simulink model "liftsubsystem"  (R2025b)
settings: Solver=VariableStepAuto  StartTime=0.0  StopTime=10  RelTol=1e-3
values from neighbouring files (symbols this model uses):
  N = 20    [ocp_arm.m]
undefined symbols (not defined in the file or in its folder): lx, ly, lz, M, m_w, X, Y, Z
libraries: sm_lib x138, nesl_utility x30, sharedTrackingLibrary x6, slpidlib x3, simulink x3, eeSlidingModeController x1, robotcorelib x1
(part 1 of 4)
settings Model: Creator=itsan  LastModifiedBy=itsan

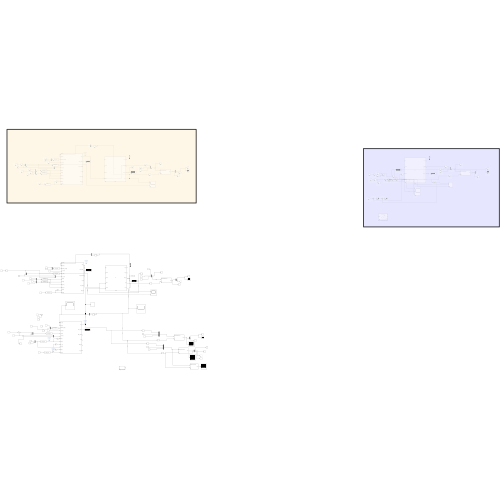
[thumbnail: Simulink's stored preview of the top-level diagram]
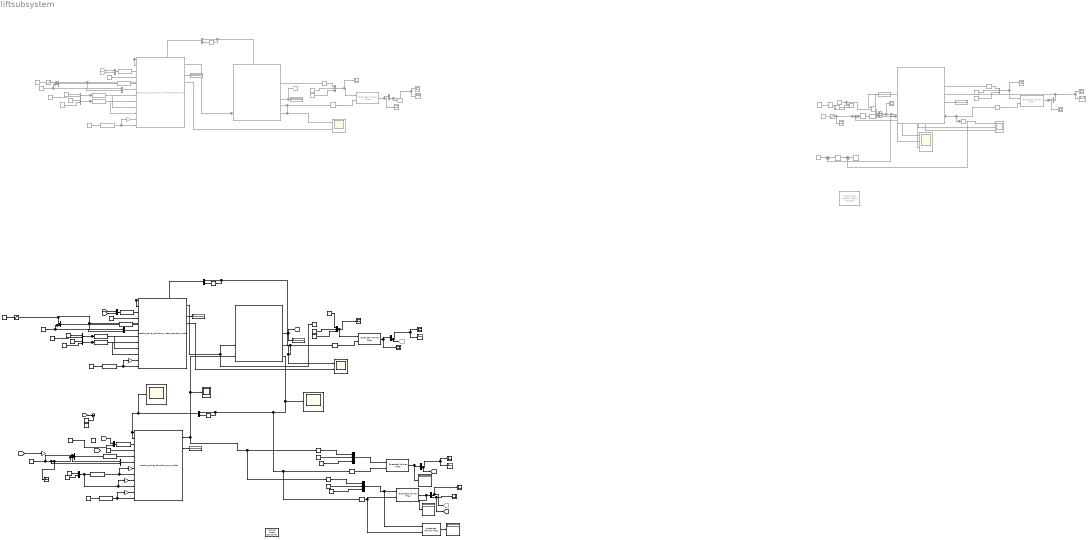
== system liftsubsystem ==
  note: Lift
  Constant : Constant  Commented=on  Value=0.5
  Constant1 : Constant  Commented=on  Value=9.81
  Constant10 : Constant  Commented=on  Value=0.01
  Constant11 : Constant  Commented=on  Value=0.5
  Constant12 : Constant  Commented=on  Value=0.8
  Constant13 : Constant  Commented=on  Value=0
  Constant14 : Constant  Commented=on  Value=150
  Constant{15,26,34..35} (4 alike) : Constant  Value=0.01
  Constant16 : Constant  Value=0.5
  Constant17 : Constant  Value=0.8
  Constant18 : Constant  Value=0
  Constant19 : Constant  Value=150
  Constant2 : Constant  Commented=on  Value=12
  Constant20 : Constant  Value=[0 0 0]
  Constant21 : Constant  Value=-0.5
  Constant22 : Constant  Value=0
  Constant23 : Constant  Value=0.43
  Constant24 : Constant  Value=0.5
  Constant25 : Constant  Value=0.5
  Constant27 : Constant  Value=100
  Constant28 : Constant  Value=[0 0 0]
  Constant29 : Constant  Value=7
  Constant3 : Constant  Commented=on  Value=0.43
  Constant30 : Constant  Value=0
  Constant31 : Constant  Value=0.4
  Constant{32..33,36..37} (4 alike) : Constant  Value=5
  Constant4 : Constant  Commented=on  Value=0.01
  Constant5 : Constant  Commented=on  Value=0.43
  Constant6 : Constant  Commented=on  Value=[0 0 0]
  Constant7 : Constant  Commented=on  Value=-0.5
  Constant8 : Constant  Commented=on  Value=0
  Constant9 : Constant  Commented=on  Value=0.43
  Cos : Trigonometry  Commented=on  Operator=cos
  Demux : Demux  Commented=on  Outputs=3
  Demux1 : Demux  Commented=on  Outputs=3
  Demux2 : Demux  Outputs=3
  Demux3 : Demux  Outputs=3
  Demux4 : Demux
  Derivative : Derivative  Commented=on
  Derivative1 : Derivative  Commented=on
  Derivative2 : Derivative
  Derivative3 : Derivative
  Display{,1..5} (6 alike) : Display  Commented=on
  Display{6..13} (8 alike) : Display
  Divide : Product  Commented=on  Inputs=***
  Divide1 : Product  Commented=on  Inputs=**
  Extended Kalman Filter : sharedTrackingLibrary/Extended Kalman Filter  Commented=on  StateTransitionFcn=myStateTransitionFcn  HasStateTransitionJacobianFcn=off  HasAdditiveProcessNoise=Additive  ProcessNoise=diag([1e-6, 1e-4, 1e-8])  HasTimeVaryingProcessNoise=off  HasStateTransitionFcnExtraArgument=1  InitialState=[0; 0; 10]  InitialStateCovariance=diag([1e-2, 1e-2, 100])  MeasurementFcn1=myMeasurementFcn  HasMeasurementJacobianFcn1=off  HasMeasurementEnablePort1=off  HasAdditiveMeasurementNoise1=Additive  MeasurementNoise1=diag([1e-2])  HasTimeVaryingMeasurementNoise1=off  HasMeasurementFcnExtraArgument1=0  HasMeasurementWrapping1=off  MeasurementFcn2=myMeasurementFcn  HasMeasurementJacobianFcn2=off  HasMeasurementEnablePort2=off  HasAdditiveMeasurementNoise2=Additive  MeasurementNoise2=1  HasTimeVaryingMeasurementNoise2=off  HasMeasurementFcnExtraArgument2=0  HasMeasurementWrapping2=off  MeasurementFcn3=myMeasurementFcn  HasMeasurementJacobianFcn3=off  HasMeasurementEnablePort3=off  HasAdditiveMeasurementNoise3=Additive  MeasurementNoise3=1  HasTimeVaryingMeasurementNoise3=off  HasMeasurementFcnExtraArgument3=0  HasMeasurementWrapping3=off  MeasurementFcn4=myMeasurementFcn  HasMeasurementJacobianFcn4=off  HasMeasurementEnablePort4=off  HasAdditiveMeasurementNoise4=Additive  MeasurementNoise4=1  HasTimeVaryingMeasurementNoise4=off  HasMeasurementFcnExtraArgument4=0  HasMeasurementWrapping4=off  MeasurementFcn5=myMeasurementFcn  HasMeasurementJacobianFcn5=off  HasMeasurementEnablePort5=off  HasAdditiveMeasurementNoise5=Additive  MeasurementNoise5=1  HasTimeVaryingMeasurementNoise5=off  HasMeasurementFcnExtraArgument5=0  HasMeasurementWrapping5=off  EnableMultirate=off  StateTransitionFcnSampleTime=1  MeasurementFcn1SampleTime=1  MeasurementFcn2SampleTime=1  MeasurementFcn3SampleTime=1  MeasurementFcn4SampleTime=1  MeasurementFcn5SampleTime=1  UseCurrentEstimator=on  OutputStateCovariance=off  DataType=double  SampleTime=0.01  NumberOfMeasurements=1
  Extended Kalman Filter1 : sharedTrackingLibrary/Extended Kalman Filter  Commented=on  StateTransitionFcn=myStateTransitionFcn  HasStateTransitionJacobianFcn=off  HasAdditiveProcessNoise=Additive  ProcessNoise=diag([1e-6, 1e-4, 1e-8])  HasTimeVaryingProcessNoise=off  HasStateTransitionFcnExtraArgument=1  InitialState=[0; 0; 10]  InitialStateCovariance=diag([1e-2, 1e-2, 100])  MeasurementFcn1=myMeasurementFcn  HasMeasurementJacobianFcn1=off  HasMeasurementEnablePort1=off  HasAdditiveMeasurementNoise1=Additive  MeasurementNoise1=diag([1e-2])  HasTimeVaryingMeasurementNoise1=off  HasMeasurementFcnExtraArgument1=0  HasMeasurementWrapping1=off  MeasurementFcn2=myMeasurementFcn  HasMeasurementJacobianFcn2=off  HasMeasurementEnablePort2=off  HasAdditiveMeasurementNoise2=Additive  MeasurementNoise2=1  HasTimeVaryingMeasurementNoise2=off  HasMeasurementFcnExtraArgument2=0  HasMeasurementWrapping2=off  MeasurementFcn3=myMeasurementFcn  HasMeasurementJacobianFcn3=off  HasMeasurementEnablePort3=off  HasAdditiveMeasurementNoise3=Additive  MeasurementNoise3=1  HasTimeVaryingMeasurementNoise3=off  HasMeasurementFcnExtraArgument3=0  HasMeasurementWrapping3=off  MeasurementFcn4=myMeasurementFcn  HasMeasurementJacobianFcn4=off  HasMeasurementEnablePort4=off  HasAdditiveMeasurementNoise4=Additive  MeasurementNoise4=1  HasTimeVaryingMeasurementNoise4=off  HasMeasurementFcnExtraArgument4=0  HasMeasurementWrapping4=off  MeasurementFcn5=myMeasurementFcn  HasMeasurementJacobianFcn5=off  HasMeasurementEnablePort5=off  HasAdditiveMeasurementNoise5=Additive  MeasurementNoise5=1  HasTimeVaryingMeasurementNoise5=off  HasMeasurementFcnExtraArgument5=0  HasMeasurementWrapping5=off  EnableMultirate=off  StateTransitionFcnSampleTime=1  MeasurementFcn1SampleTime=1  MeasurementFcn2SampleTime=1  MeasurementFcn3SampleTime=1  MeasurementFcn4SampleTime=1  MeasurementFcn5SampleTime=1  UseCurrentEstimator=on  OutputStateCovariance=off  DataType=double  SampleTime=0.01  NumberOfMeasurements=1
  Extended Kalman Filter2 : sharedTrackingLibrary/Extended Kalman Filter  StateTransitionFcn=liftStateTransitionFcn  HasStateTransitionJacobianFcn=off  HasAdditiveProcessNoise=Additive  ProcessNoise=diag([1e-6, 1e-4, 1e-8])  HasTimeVaryingProcessNoise=off  HasStateTransitionFcnExtraArgument=1  InitialState=[0; 0; 10]  InitialStateCovariance=diag([1e-2, 1e-2, 100])  MeasurementFcn1=liftMeasurementFcn  HasMeasurementJacobianFcn1=off  HasMeasurementEnablePort1=off  HasAdditiveMeasurementNoise1=Additive  MeasurementNoise1=diag([1e-2])  HasTimeVaryingMeasurementNoise1=off  HasMeasurementFcnExtraArgument1=0  HasMeasurementWrapping1=off  MeasurementFcn2=myMeasurementFcn  HasMeasurementJacobianFcn2=off  HasMeasurementEnablePort2=off  HasAdditiveMeasurementNoise2=Additive  MeasurementNoise2=1  HasTimeVaryingMeasurementNoise2=off  HasMeasurementFcnExtraArgument2=0  HasMeasurementWrapping2=off  MeasurementFcn3=myMeasurementFcn  HasMeasurementJacobianFcn3=off  HasMeasurementEnablePort3=off  HasAdditiveMeasurementNoise3=Additive  MeasurementNoise3=1  HasTimeVaryingMeasurementNoise3=off  HasMeasurementFcnExtraArgument3=0  HasMeasurementWrapping3=off  MeasurementFcn4=myMeasurementFcn  HasMeasurementJacobianFcn4=off  HasMeasurementEnablePort4=off  HasAdditiveMeasurementNoise4=Additive  MeasurementNoise4=1  HasTimeVaryingMeasurementNoise4=off  HasMeasurementFcnExtraArgument4=0  HasMeasurementWrapping4=off  MeasurementFcn5=myMeasurementFcn  HasMeasurementJacobianFcn5=off  HasMeasurementEnablePort5=off  HasAdditiveMeasurementNoise5=Additive  MeasurementNoise5=1  HasTimeVaryingMeasurementNoise5=off  HasMeasurementFcnExtraArgument5=0  HasMeasurementWrapping5=off  EnableMultirate=off  StateTransitionFcnSampleTime=1  MeasurementFcn1SampleTime=1  MeasurementFcn2SampleTime=1  MeasurementFcn3SampleTime=1  MeasurementFcn4SampleTime=1  MeasurementFcn5SampleTime=1  UseCurrentEstimator=on  OutputStateCovariance=off  DataType=double  SampleTime=0.01  NumberOfMeasurements=1
  Extended Kalman Filter3 : sharedTrackingLibrary/Extended Kalman Filter  StateTransitionFcn=armStateTransitionFcn  HasStateTransitionJacobianFcn=off  HasAdditiveProcessNoise=Additive  ProcessNoise=diag([1e-8, 1e-6,1e-10])  HasTimeVaryingProcessNoise=off  HasStateTransitionFcnExtraArgument=1  InitialState=[0;0;0.3]  InitialStateCovariance=diag([1e-4, 1e-4,100])  MeasurementFcn1=armMeasurementFcn  HasMeasurementJacobianFcn1=off  HasMeasurementEnablePort1=off  HasAdditiveMeasurementNoise1=Additive  MeasurementNoise1=1e-4  HasTimeVaryingMeasurementNoise1=off  HasMeasurementFcnExtraArgument1=0  HasMeasurementWrapping1=off  MeasurementFcn2=myMeasurementFcn  HasMeasurementJacobianFcn2=off  HasMeasurementEnablePort2=off  HasAdditiveMeasurementNoise2=Additive  MeasurementNoise2=1  HasTimeVaryingMeasurementNoise2=off  HasMeasurementFcnExtraArgument2=0  HasMeasurementWrapping2=off  MeasurementFcn3=myMeasurementFcn  HasMeasurementJacobianFcn3=off  HasMeasurementEnablePort3=off  HasAdditiveMeasurementNoise3=Additive  MeasurementNoise3=1  HasTimeVaryingMeasurementNoise3=off  HasMeasurementFcnExtraArgument3=0  HasMeasurementWrapping3=off  MeasurementFcn4=myMeasurementFcn  HasMeasurementJacobianFcn4=off  HasMeasurementEnablePort4=off  HasAdditiveMeasurementNoise4=Additive  MeasurementNoise4=1  HasTimeVaryingMeasurementNoise4=off  HasMeasurementFcnExtraArgument4=0  HasMeasurementWrapping4=off  MeasurementFcn5=myMeasurementFcn  HasMeasurementJacobianFcn5=off  HasMeasurementEnablePort5=off  HasAdditiveMeasurementNoise5=Additive  MeasurementNoise5=1  HasTimeVaryingMeasurementNoise5=off  HasMeasurementFcnExtraArgument5=0  HasMeasurementWrapping5=off  EnableMultirate=off  StateTransitionFcnSampleTime=1  MeasurementFcn1SampleTime=1  MeasurementFcn2SampleTime=1  MeasurementFcn3SampleTime=1  MeasurementFcn4SampleTime=1  MeasurementFcn5SampleTime=1  UseCurrentEstimator=on  OutputStateCovariance=off  DataType=double  SampleTime=0.01  NumberOfMeasurements=1
  Extended Kalman Filter5 : sharedTrackingLibrary/Extended Kalman Filter  StateTransitionFcn=armMassStateTransitionFcn  HasStateTransitionJacobianFcn=off  HasAdditiveProcessNoise=Additive  ProcessNoise=diag([1e-8, 1e-6,1e-10,1e-10])  HasTimeVaryingProcessNoise=off  HasStateTransitionFcnExtraArgument=1  InitialState=[0;0;0.3;5]  InitialStateCovariance=diag([1e-4, 1e-4,100,100])  MeasurementFcn1=armMeasurementFcn  HasMeasurementJacobianFcn1=off  HasMeasurementEnablePort1=off  HasAdditiveMeasurementNoise1=Additive  MeasurementNoise1=1e-4  HasTimeVaryingMeasurementNoise1=off  HasMeasurementFcnExtraArgument1=0  HasMeasurementWrapping1=off  MeasurementFcn2=myMeasurementFcn  HasMeasurementJacobianFcn2=off  HasMeasurementEnablePort2=off  HasAdditiveMeasurementNoise2=Additive  MeasurementNoise2=1  HasTimeVaryingMeasurementNoise2=off  HasMeasurementFcnExtraArgument2=0  HasMeasurementWrapping2=off  MeasurementFcn3=myMeasurementFcn  HasMeasurementJacobianFcn3=off  HasMeasurementEnablePort3=off  HasAdditiveMeasurementNoise3=Additive  MeasurementNoise3=1  HasTimeVaryingMeasurementNoise3=off  HasMeasurementFcnExtraArgument3=0  HasMeasurementWrapping3=off  MeasurementFcn4=myMeasurementFcn  HasMeasurementJacobianFcn4=off  HasMeasurementEnablePort4=off  HasAdditiveMeasurementNoise4=Additive  MeasurementNoise4=1  HasTimeVaryingMeasurementNoise4=off  HasMeasurementFcnExtraArgument4=0  HasMeasurementWrapping4=off  MeasurementFcn5=myMeasurementFcn  HasMeasurementJacobianFcn5=off  HasMeasurementEnablePort5=off  HasAdditiveMeasurementNoise5=Additive  MeasurementNoise5=1  HasTimeVaryingMeasurementNoise5=off  HasMeasurementFcnExtraArgument5=0  HasMeasurementWrapping5=off  EnableMultirate=off  StateTransitionFcnSampleTime=1  MeasurementFcn1SampleTime=1  MeasurementFcn2SampleTime=1  MeasurementFcn3SampleTime=1  MeasurementFcn4SampleTime=1  MeasurementFcn5SampleTime=1  UseCurrentEstimator=on  OutputStateCovariance=off  DataType=double  SampleTime=0.01  NumberOfMeasurements=1
  From : From  Commented=on  GotoTag=Mass
  From1 : From  Commented=on  GotoTag=Pitch
  Gain : Gain  Commented=on  Gain=-1
  Gain{1..5} (5 alike) : Gain  Gain=-1
  Goto : Goto  Commented=on  GotoTag=Mass
  Goto1 : Goto  Commented=on  GotoTag=Pitch
  Goto2 : Goto  Commented=on  GotoTag=Mass
  Goto5 : Goto  Commented=on  GotoTag=rx
  Mux{,2,5..7} (5 alike) : Mux  Commented=on  Inputs=2
  Mux1 : Mux  Commented=on  Inputs=3
  Mux{8,10,12..15,18..20} (9 alike) : Mux  Inputs=2
  Mux{9,11,16..17,21} (5 alike) : Mux  Inputs=3
  Mux3 : Mux  Commented=on  Inputs=3
  Mux4 : Mux  Commented=on  Inputs=3
  PD : slpidlib/PID Controller  Commented=on  Controller=PID  Form=Parallel  TimeDomain=Continuous-time  UseExternalTs=off  SampleTime=-1  IntegratorMethod=Forward Euler  FilterMethod=Forward Euler  ControllerParametersSource=internal  P=1  I=0.001  UseKiTs=off  D=22  UseExternalDerivativeSource=off  N=15  UseFilter=on  TunerSelectOption=Transfer Function Based (PID Tuner App)  InitialConditionSource=internal  InitialConditionForIntegrator=0  InitialConditionForFilter=0  DifferentiatorICPrevScaledInput=0  ExternalReset=none  TrackingMode=off  Kt=1  LimitOutput=on  SatLimitsSource=internal  UpperSaturationLimit=100  LowerSaturationLimit=-100  LinearizeAsGain=on  AntiWindupMode=back-calculation  Kb=3  LimitIntegrator=off  UpperIntegratorSaturationLimit=inf  LowerIntegratorSaturationLimit=-inf  POutMin=[]  POutMax=[]  IOutMin=[]  IOutMax=[]  DOutMin=[]  DOutMax=[]  NOutMin=[]  NOutMax=[]  SumOutMin=[]  SumOutMax=[]  SaturationOutMin=[]  SaturationOutMax=[]  PParamMin=[]  PParamMax=[]  IParamMin=[]  IParamMax=[]  DParamMin=[]  DParamMax=[]  NParamMin=[]  NParamMax=[]  KbParamMin=[]  KbParamMax=[]  KtParamMin=[]  KtParamMax=[]  KbOutMin=[]  KbOutMax=[]  KtOutMin=[]  KtOutMax=[]  IntegratorOutMin=[]  IntegratorOutMax=[]  FilterOutMin=[]  FilterOutMax=[]  SumI1OutMin=[]  SumI1OutMax=[]  SumI2OutMin=[]  SumI2OutMax=[]  SumI3OutMin=[]  SumI3OutMax=[]  SumI4OutMin=[]  SumI4OutMax=[]  SumDOutMin=[]  SumDOutMax=[]  DifferentiatorOutMin=[]  DifferentiatorOutMax=[]  FilterDiffOutCoefMin=[]  FilterDiffOutCoefMax=[]  ReciprocalOutMin=[]  ReciprocalOutMax=[]  SumDenOutMin=[]  SumDenOutMax=[]  SumNumOutMin=[]  SumNumOutMax=[]  DivideOutMin=[]  DivideOutMax=[]  UdiffTsProdOutMin=[]  UdiffTsProdOutMax=[]  NTsProdOutMin=[]  NTsProdOutMax=[]  UintegralTsProdOutMin=[]  UintegralTsProdOutMax=[]  UngainTsProdOutMin=[]  UngainTsProdOutMax=[]  ClampingZeroOutDataTypeStr=Inherit: Inherit via back propagation  ClampingZeroOutMin=[]  ClampingZeroOutMax=[]  FilterDenConstantOutDataTypeStr=Inherit: Inherit via back propagation  FilterDenConstantOutMin=[]  FilterDenConstantOutMax=[]  PCopyOutDataTypeStr=Inherit: Inherit via back propagation  PCopyOutMin=[]  PCopyOutMax=[]  NCopyOutDataTypeStr=Inherit: Inherit via back propagation  NCopyOutMin=[]  NCopyOutMax=[]  IntegratorContinuousStateAttributes=''  IntegratorStateMustResolveToSignalObject=off  IntegratorRTWStateStorageClass=Auto  FilterContinuousStateAttributes=''  FilterStateMustResolveToSignalObject=off  FilterRTWStateStorageClass=Auto  ParallelPVariant=InternalParameters  IdealPVariant=Disabled  IVariant=InternalParameters  DVariant=InternalParameters  IntegratorVariant=Continuous  SatVariant=Enabled  AWVariant=BackCalculation  PCopyVariant=Disabled  TRVariant=Disabled  FdbkBlocksVariant=Forward  IdealPFdbkVariant=Disabled  SatFdbkVariant=Disabled  DerivativeFilterVariant=ContFilter  NVariant=InternalParameters  NCopyVariant=Disabled  FilterICVariant=InternalICsFilter  IntegratorICVariant=InternalICs  ExternalResetVariant=Disabled  TRSumVariant=Passthrough  SumFdbkVariant=Disabled  SumVariant=Sum_PID  TsampFilterVariant=InternalTs  TsampNgainVariant=Passthrough  TsampIntegralVariant=Disabled_SignalSpec  ExternalSaturationOutDataTypeStr=Inherit: Same as second input  DerivativeSourceVariant=ErrorSignal  PreIntVariant=InternalPreInt
  PID Controller : slpidlib/PID Controller  Commented=on  Controller=PID  Form=Parallel  TimeDomain=Continuous-time  UseExternalTs=off  SampleTime=-1  IntegratorMethod=Forward Euler  FilterMethod=Forward Euler  ControllerParametersSource=internal  P=10  I=0  UseKiTs=off  D=0  UseExternalDerivativeSource=off  N=0  UseFilter=on  TunerSelectOption=Transfer Function Based (PID Tuner App)  InitialConditionSource=internal  InitialConditionForIntegrator=0  InitialConditionForFilter=0  DifferentiatorICPrevScaledInput=0  ExternalReset=none  TrackingMode=off  Kt=1  LimitOutput=on  SatLimitsSource=internal  UpperSaturationLimit=1  LowerSaturationLimit=-1  LinearizeAsGain=on  AntiWindupMode=none  Kb=1  LimitIntegrator=off  UpperIntegratorSaturationLimit=inf  LowerIntegratorSaturationLimit=-inf  POutMin=[]  POutMax=[]  IOutMin=[]  IOutMax=[]  DOutMin=[]  DOutMax=[]  NOutMin=[]  NOutMax=[]  SumOutMin=[]  SumOutMax=[]  SaturationOutMin=[]  SaturationOutMax=[]  PParamMin=[]  PParamMax=[]  IParamMin=[]  IParamMax=[]  DParamMin=[]  DParamMax=[]  NParamMin=[]  NParamMax=[]  KbParamMin=[]  KbParamMax=[]  KtParamMin=[]  KtParamMax=[]  KbOutMin=[]  KbOutMax=[]  KtOutMin=[]  KtOutMax=[]  IntegratorOutMin=[]  IntegratorOutMax=[]  FilterOutMin=[]  FilterOutMax=[]  SumI1OutMin=[]  SumI1OutMax=[]  SumI2OutMin=[]  SumI2OutMax=[]  SumI3OutMin=[]  SumI3OutMax=[]  SumI4OutMin=[]  SumI4OutMax=[]  SumDOutMin=[]  SumDOutMax=[]  DifferentiatorOutMin=[]  DifferentiatorOutMax=[]  FilterDiffOutCoefMin=[]  FilterDiffOutCoefMax=[]  ReciprocalOutMin=[]  ReciprocalOutMax=[]  SumDenOutMin=[]  SumDenOutMax=[]  SumNumOutMin=[]  SumNumOutMax=[]  DivideOutMin=[]  DivideOutMax=[]  UdiffTsProdOutMin=[]  UdiffTsProdOutMax=[]  NTsProdOutMin=[]  NTsProdOutMax=[]  UintegralTsProdOutMin=[]  UintegralTsProdOutMax=[]  UngainTsProdOutMin=[]  UngainTsProdOutMax=[]  ClampingZeroOutDataTypeStr=Inherit: Inherit via back propagation  ClampingZeroOutMin=[]  ClampingZeroOutMax=[]  FilterDenConstantOutDataTypeStr=Inherit: Inherit via back propagation  FilterDenConstantOutMin=[]  FilterDenConstantOutMax=[]  PCopyOutDataTypeStr=Inherit: Inherit via back propagation  PCopyOutMin=[]  PCopyOutMax=[]  NCopyOutDataTypeStr=Inherit: Inherit via back propagation  NCopyOutMin=[]  NCopyOutMax=[]  IntegratorContinuousStateAttributes=''  IntegratorStateMustResolveToSignalObject=off  IntegratorRTWStateStorageClass=Auto  FilterContinuousStateAttributes=''  FilterStateMustResolveToSignalObject=off  FilterRTWStateStorageClass=Auto  ParallelPVariant=InternalParameters  IdealPVariant=Disabled  IVariant=InternalParameters  DVariant=InternalParameters  IntegratorVariant=Continuous  SatVariant=Enabled  AWVariant=Passthrough  PCopyVariant=Disabled  TRVariant=Disabled  FdbkBlocksVariant=Forward  IdealPFdbkVariant=Disabled  SatFdbkVariant=Disabled  DerivativeFilterVariant=ContFilter  NVariant=InternalParameters  NCopyVariant=Disabled  FilterICVariant=InternalICsFilter  IntegratorICVariant=InternalICs  ExternalResetVariant=Disabled  TRSumVariant=Passthrough  SumFdbkVariant=Disabled  SumVariant=Sum_PID  TsampFilterVariant=InternalTs  TsampNgainVariant=Passthrough  TsampIntegralVariant=Disabled_SignalSpec  ExternalSaturationOutDataTypeStr=Inherit: Same as second input  DerivativeSourceVariant=ErrorSignal  PreIntVariant=InternalPreInt
  PID Controller1 : slpidlib/PID Controller  Commented=on  Controller=PID  Form=Parallel  TimeDomain=Continuous-time  UseExternalTs=off  SampleTime=-1  IntegratorMethod=Forward Euler  FilterMethod=Forward Euler  ControllerParametersSource=internal  P=10  I=4  UseKiTs=off  D=0  UseExternalDerivativeSource=off  N=0  UseFilter=on  TunerSelectOption=Transfer Function Based (PID Tuner App)  InitialConditionSource=internal  InitialConditionForIntegrator=0  InitialConditionForFilter=0  DifferentiatorICPrevScaledInput=0  ExternalReset=none  TrackingMode=off  Kt=1  LimitOutput=on  SatLimitsSource=internal  UpperSaturationLimit=1  LowerSaturationLimit=-1  LinearizeAsGain=on  AntiWindupMode=none  Kb=1  LimitIntegrator=off  UpperIntegratorSaturationLimit=inf  LowerIntegratorSaturationLimit=-inf  POutMin=[]  POutMax=[]  IOutMin=[]  IOutMax=[]  DOutMin=[]  DOutMax=[]  NOutMin=[]  NOutMax=[]  SumOutMin=[]  SumOutMax=[]  SaturationOutMin=[]  SaturationOutMax=[]  PParamMin=[]  PParamMax=[]  IParamMin=[]  IParamMax=[]  DParamMin=[]  DParamMax=[]  NParamMin=[]  NParamMax=[]  KbParamMin=[]  KbParamMax=[]  KtParamMin=[]  KtParamMax=[]  KbOutMin=[]  KbOutMax=[]  KtOutMin=[]  KtOutMax=[]  IntegratorOutMin=[]  IntegratorOutMax=[]  FilterOutMin=[]  FilterOutMax=[]  SumI1OutMin=[]  SumI1OutMax=[]  SumI2OutMin=[]  SumI2OutMax=[]  SumI3OutMin=[]  SumI3OutMax=[]  SumI4OutMin=[]  SumI4OutMax=[]  SumDOutMin=[]  SumDOutMax=[]  DifferentiatorOutMin=[]  DifferentiatorOutMax=[]  FilterDiffOutCoefMin=[]  FilterDiffOutCoefMax=[]  ReciprocalOutMin=[]  ReciprocalOutMax=[]  SumDenOutMin=[]  SumDenOutMax=[]  SumNumOutMin=[]  SumNumOutMax=[]  DivideOutMin=[]  DivideOutMax=[]  UdiffTsProdOutMin=[]  UdiffTsProdOutMax=[]  NTsProdOutMin=[]  NTsProdOutMax=[]  UintegralTsProdOutMin=[]  UintegralTsProdOutMax=[]  UngainTsProdOutMin=[]  UngainTsProdOutMax=[]  ClampingZeroOutDataTypeStr=Inherit: Inherit via back propagation  ClampingZeroOutMin=[]  ClampingZeroOutMax=[]  FilterDenConstantOutDataTypeStr=Inherit: Inherit via back propagation  FilterDenConstantOutMin=[]  FilterDenConstantOutMax=[]  PCopyOutDataTypeStr=Inherit: Inherit via back propagation  PCopyOutMin=[]  PCopyOutMax=[]  NCopyOutDataTypeStr=Inherit: Inherit via back propagation  NCopyOutMin=[]  NCopyOutMax=[]  IntegratorContinuousStateAttributes=''  IntegratorStateMustResolveToSignalObject=off  IntegratorRTWStateStorageClass=Auto  FilterContinuousStateAttributes=''  FilterStateMustResolveToSignalObject=off  FilterRTWStateStorageClass=Auto  ParallelPVariant=InternalParameters  IdealPVariant=Disabled  IVariant=InternalParameters  DVariant=InternalParameters  IntegratorVariant=Continuous  SatVariant=Enabled  AWVariant=Passthrough  PCopyVariant=Disabled  TRVariant=Disabled  FdbkBlocksVariant=Forward  IdealPFdbkVariant=Disabled  SatFdbkVariant=Disabled  DerivativeFilterVariant=ContFilter  NVariant=InternalParameters  NCopyVariant=Disabled  FilterICVariant=InternalICsFilter  IntegratorICVariant=InternalICs  ExternalResetVariant=Disabled  TRSumVariant=Passthrough  SumFdbkVariant=Disabled  SumVariant=Sum_PID  TsampFilterVariant=InternalTs  TsampNgainVariant=Passthrough  TsampIntegralVariant=Disabled_SignalSpec  ExternalSaturationOutDataTypeStr=Inherit: Same as second input  DerivativeSourceVariant=ErrorSignal  PreIntVariant=InternalPreInt
  Plant1 : Subsystem  Commented=on
      mask Display: image('plant.png');
  Plant2 : Subsystem  Commented=on
      mask Display: image('plant.png');
  Plant3 : Subsystem
      mask Display: image('plant.png');
  Ramp : simulink/Sources/Ramp  Commented=on  slope=0.5  start=0  InitialOutput=0
  Ramp1 : simulink/Sources/Ramp  Commented=on  slope=1  start=0  InitialOutput=0
  Ramp3 : simulink/Sources/Ramp  slope=1  start=0  InitialOutput=0
  S-Function : S-Function  Commented=on  FunctionName=repmat_sfun  Parameters=N+1  SFunctionDeploymentMode=off  EnableBusSupport=off
  S-Function1 : S-Function  Commented=on  FunctionName=acados_solver_sfunction_linear_actuator_model  SFunctionDeploymentMode=off  EnableBusSupport=off
      mask Display:
      | % from the make_sfun file
      | global sfun_input_names sfun_output_names
      | for i = 1:length(sfun_input_names)
      | 	port_label('input', i, sfun_input_names{i})
      | end
      | for i = 1:length(sfun_output_names)
      | 	port_label('output', i, sfun_output_names{i})
      | end
  S-Function{8..10,12,16} (5 alike) : S-Function  FunctionName=repmat_sfun  Parameters=N-1  SFunctionDeploymentMode=off  EnableBusSupport=off
  S-Function11 : S-Function  FunctionName=repmat_sfun  Parameters=N  SFunctionDeploymentMode=off  EnableBusSupport=off
  S-Function13 : S-Function  FunctionName=repmat_sfun  Parameters=N  SFunctionDeploymentMode=off  EnableBusSupport=off
  S-Function14 : S-Function  FunctionName=repmat_sfun  Parameters=N+1  SFunctionDeploymentMode=off  EnableBusSupport=off
  S-Function15 : S-Function  FunctionName=acados_solver_sfunction_arm_model  SFunctionDeploymentMode=off  EnableBusSupport=off
      mask Display:
      | % from the make_sfun file
      | global sfun_input_names sfun_output_names
      | for i = 1:length(sfun_input_names)
      | 	port_label('input', i, sfun_input_names{i})
      | end
      | for i = 1:length(sfun_output_names)
      | 	port_label('output', i, sfun_output_names{i})
      | end
  S-Function2 : S-Function  Commented=on  FunctionName=repmat_sfun  Parameters=N-1  SFunctionDeploymentMode=off  EnableBusSupport=off
  S-Function3 : S-Function  Commented=on  FunctionName=repmat_sfun  Parameters=N-1  SFunctionDeploymentMode=off  EnableBusSupport=off
  S-Function4 : S-Function  Commented=on  FunctionName=repmat_sfun  Parameters=N-1  SFunctionDeploymentMode=off  EnableBusSupport=off
  S-Function5 : S-Function  Commented=on  FunctionName=repmat_sfun  Parameters=N  SFunctionDeploymentMode=off  EnableBusSupport=off
  S-Function6 : S-Function  FunctionName=repmat_sfun  Parameters=N+1  SFunctionDeploymentMode=off  EnableBusSupport=off
  S-Function7 : S-Function  FunctionName=acados_solver_sfunction_linear_actuator_model  SFunctionDeploymentMode=off  EnableBusSupport=off
      mask Display:
      | % from the make_sfun file
      | global sfun_input_names sfun_output_names
      | for i = 1:length(sfun_input_names)
      | 	port_label('input', i, sfun_input_names{i})
      | end
      | for i = 1:length(sfun_output_names)
      | 	port_label('output', i, sfun_output_names{i})
      | end
  Saturation : Saturate  Commented=on
  Saturation1 : Saturate  Commented=on
  Saturation3 : Saturate  UpperLimit=0.1
  Scope{,2..4,6,9..10,13} (8 alike) : Scope  Commented=on
      Scope settings: ActiveDisplayYMinimum=117.38726606594429  ActiveDisplayYMaximum=117.96497291719386
      Scope10 settings: ActiveDisplayYMinimum=10.368033685081326  ActiveDisplayYMaximum=13.754521835601309  DataLoggingVariableName=ScopeData7
      Scope13 settings: ActiveDisplayYMinimum=-23.500486572497707  ActiveDisplayYMaximum=44.300288166456191  DataLoggingVariableName=ScopeData10
      Scope2 settings: ActiveDisplayYMinimum=-23.500486572497707  ActiveDisplayYMaximum=44.300288166456191  DataLoggingVariableName=ScopeData2
      Scope3 settings: ActiveDisplayYMinimum=9.4746445379021456  ActiveDisplayYMaximum=14.728199158880699  DataLoggingVariableName=ScopeData3
      Scope4 settings: ActiveDisplayYMinimum=-0.93767561156709411  ActiveDisplayYMaximum=3.3247649685442195  DataLoggingVariableName=ScopeData4
      Scope6 settings: ActiveDisplayYMinimum=-23.500486572497707  ActiveDisplayYMaximum=44.300288166456191  DataLoggingVariableName=ScopeData6
      Scope9 settings: ActiveDisplayYMinimum=-23.500486572497707  ActiveDisplayYMaximum=44.300288166456191  DataLoggingVariableName=ScopeData13
  Scope1 : Scope  Commented=on  NumInputPorts=3
      settings: ActiveDisplayYMinimum=-0.20308839711342824  ActiveDisplayYMaximum=1.2259812299014095
  Scope{8,11,14..21} (10 alike) : Scope
      Scope11 settings: ActiveDisplayYMinimum=-23.500486572497707  ActiveDisplayYMaximum=44.300288166456191  DataLoggingVariableName=ScopeData9
      Scope14 settings: ActiveDisplayYMinimum=-23.500486572497707  ActiveDisplayYMaximum=44.300288166456191  DataLoggingVariableName=ScopeData12
      Scope15 settings: ActiveDisplayYMinimum=-1  ActiveDisplayYMaximum=1  DataLoggingVariableName=ScopeData21
      Scope16 settings: ActiveDisplayYMinimum=-0.71979355278070756  ActiveDisplayYMaximum=3.517359474034798  DataLoggingVariableName=ScopeData22
      Scope17 settings: ActiveDisplayYMinimum=-6.4823784268845435  ActiveDisplayYMaximum=-3.5314469973157538  DataLoggingVariableName=ScopeData23
      Scope18 settings: ActiveDisplayYMinimum=-0.06438015181759206  ActiveDisplayYMaximum=0.57942136635832864  DataLoggingVariableName=ScopeData24
      Scope19 settings: ActiveDisplayYMinimum=-2.1280646608999834  ActiveDisplayYMaximum=0.5697849623222202  DataLoggingVariableName=ScopeData25
      Scope20 settings: ActiveDisplayYMinimum=-0.38236324419750722  ActiveDisplayYMaximum=1.1874760943553313  DataLoggingVariableName=ScopeData26
      Scope21 settings: ActiveDisplayYMinimum=1.9443012041456544  ActiveDisplayYMaximum=7.9947731693161028  DataLoggingVariableName=ScopeData27
      Scope8 settings: ActiveDisplayYMinimum=1.7628570115484123  ActiveDisplayYMaximum=12.261814228718583  DataLoggingVariableName=ScopeData19
  Scope12 : Scope  NumInputPorts=2
      settings: ActiveDisplayYMinimum=-0.12609078655591466  ActiveDisplayYMaximum=0.56374645055007666  DataLoggingVariableName=ScopeData11
  Scope5 : Scope  Commented=on  NumInputPorts=3
      settings: ActiveDisplayYMinimum=-3.3927367175447758  ActiveDisplayYMaximum=3.8241131199467557  DataLoggingVariableName=ScopeData5
  Scope7 : Scope  Commented=on  NumInputPorts=2
      settings: ActiveDisplayYMinimum=-0.12609078655591466  ActiveDisplayYMaximum=0.56374645055007666  DataLoggingVariableName=ScopeData8
  Signal Specification : SignalSpecification  Commented=on  OutDataTypeStr=double  Dimensions=1
  Sliding Mode Controller : eeSlidingModeController/Sliding Mode Controller  lambda=1  h=0.2  up=10  lo=-10  Ts=-1
      settings: LibrarySourceBlock=ee_sl_lib/General Control/Sliding Mode Controller
  Sum : Sum  Commented=on  Inputs=|+-
  Sum1 : Sum  Commented=on  Inputs=+|+
  Sum2 : Sum  Commented=on  Inputs=|+-
  Sum3 : Sum  Commented=on  Inputs=|+-
  Sum4 : Sum  Inputs=|+-
  Trapezoidal Velocity Profile Trajectory : robotcorelib/Trapezoidal Velocity Profile Trajectory  Commented=on  WaypointSource=Internal  Waypoints=[ 0, -0.5, -1; 0, 0.5, 1 ]  NumParams=0  Parameter1=Peak Velocity  Parameter2=End Time  ParameterSource=Internal  PeakVelocity=[ 2; 2 ]  Acceleration=[ 1; 2 ]  EndTime=[ 1; 1 ]  AccelTime=[ 1; 2 ]  SimulateUsing=Code generation
  Unscented Kalman Filter1 : sharedTrackingLibrary/Unscented Kalman Filter  StateTransitionFcn=armMassStateTransitionUKF  HasAdditiveProcessNoise=Additive  ProcessNoise=diag([1e-8, 1e-6,1e-3])  HasTimeVaryingProcessNoise=off  HasStateTransitionFcnExtraArgument=1  InitialState=[0;0;0.5]  InitialStateCovariance=diag([1e-4, 1e-3, 0.2])  Alpha=1e-3  Beta=2  Kappa=0  MeasurementFcn1=armMeasurementUKF  HasMeasurementEnablePort1=off  HasAdditiveMeasurementNoise1=Additive  MeasurementNoise1=1e-4  HasTimeVaryingMeasurementNoise1=off  HasMeasurementFcnExtraArgument1=0  HasMeasurementWrapping1=off  MeasurementFcn2=myMeasurementFcn  HasMeasurementEnablePort2=off  HasAdditiveMeasurementNoise2=Additive  MeasurementNoise2=1  HasTimeVaryingMeasurementNoise2=off  HasMeasurementFcnExtraArgument2=0  HasMeasurementWrapping2=off  MeasurementFcn3=myMeasurementFcn  HasMeasurementEnablePort3=off  HasAdditiveMeasurementNoise3=Additive  MeasurementNoise3=1  HasTimeVaryingMeasurementNoise3=off  HasMeasurementFcnExtraArgument3=0  HasMeasurementWrapping3=off  MeasurementFcn4=myMeasurementFcn  HasMeasurementEnablePort4=off  HasAdditiveMeasurementNoise4=Additive  MeasurementNoise4=1  HasTimeVaryingMeasurementNoise4=off  HasMeasurementFcnExtraArgument4=0  HasMeasurementWrapping4=off  MeasurementFcn5=myMeasurementFcn  HasMeasurementEnablePort5=off  HasAdditiveMeasurementNoise5=Additive  MeasurementNoise5=1  HasTimeVaryingMeasurementNoise5=off  HasMeasurementFcnExtraArgument5=0  HasMeasurementWrapping5=off  EnableMultirate=off  StateTransitionFcnSampleTime=1  MeasurementFcn1SampleTime=1  MeasurementFcn2SampleTime=1  MeasurementFcn3SampleTime=1  MeasurementFcn4SampleTime=1  MeasurementFcn5SampleTime=1  UseCurrentEstimator=on  OutputStateCovariance=off  DataType=double  SampleTime=0.01  NumberOfMeasurements=1
      settings: LibrarySourceBlock=cstblocks/State Estimation/Unscented Kalman Filter
  Zero-Order Hold{,5..9} (6 alike) : ZeroOrderHold  SampleTime=0.01
  Zero-Order Hold{1..4} (4 alike) : ZeroOrderHold  Commented=on  SampleTime=0.01
  wires:
  Sum/1 -> PID Controller/1
  Constant/1 -> Sum/1
  Constant1/1 -> Divide1/2, Divide/1
  Derivative/1 -> Sum2/2
  PID Controller/1 -> Sum2/1
  Sum2/1 -> PID Controller1/1
  Extended Kalman Filter/1 -> Scope2/1, Demux/1
  Plant1/4(lift_pos) -> Sum3/2, Sum/2, Scope5/3, Zero-Order Hold2/1, Derivative/1, Scope1/1
  Demux/3 -> Scope3/1, Display/1, Divide1/1
  Saturation/1 -> Scope1/2, Sum3/1, Scope4/1  "ref"
  Constant4/1 -> Mux3/2
  Sum1/1 -> Scope/1, Scope5/1, Zero-Order Hold1/1, Plant1/4(liftForce), Display2/1  "utotal"
  Signal Specification/1 -> Scope5/2, Sum1/2  "upid"
  Ramp/1 -> Saturation/1
  PD/1 -> Signal Specification/1
  Sum3/1 -> Scope1/3, PD/1  "error"
  Constant3/1 -> Mux3/3
  Zero-Order Hold1/1 -> Mux3/1
  Zero-Order Hold2/1 -> Extended Kalman Filter/2
  Mux3/1 -> Extended Kalman Filter/1, Scope6/1  "inputs"
  Constant2/1 -> Divide/3
  Cos/1 -> Divide/2
  Plant1/3(pitch_angle) -> Display1/1  "pitch_angle"
  Constant5/1 -> Cos/1
  Divide1/1 -> Sum1/1
  Constant10/1 -> Mux1/2
  Plant2/4(lift_pos) -> Scope7/1, Zero-Order Hold4/1, Derivative1/1, Mux/1
  Extended Kalman Filter1/1 -> Scope9/1, Demux1/1
  Mux1/1 -> Extended Kalman Filter1/1, Scope13/1  "inputs"
  Zero-Order Hold4/1 -> Extended Kalman Filter1/2
  Demux1/3 -> Goto/1, Scope10/1, Display3/1
  Zero-Order Hold3/1 -> Mux1/1
  Plant2/3(pitch_angle) -> Goto1/1, Display4/1  "pitch_angle"
  Constant9/1 -> Mux1/3
  Derivative1/1 -> Mux/2
  Mux/1 -> S-Function1/2, S-Function1/1
  S-Function1/1 -> Zero-Order Hold3/1, Plant2/4(liftForce)  "u"
  S-Function1/2 -> Display5/1
  Constant6/1 -> S-Function1/4
  S-Function/1 -> S-Function1/3
  Mux2/1 -> S-Function/1
  S-Function2/1 -> S-Function1/5
  Ramp1/1 -> Saturation1/1
  Saturation1/1 -> Mux7/1, Scope7/2, Mux4/1
  Constant8/1 -> Mux7/2, Mux4/3, Mux4/2
  Mux4/1 -> S-Function2/1
  S-Function3/1 -> S-Function1/7
  Constant7/1 -> Mux5/2
  Mux5/1 -> S-Function1/9, S-Function3/1
  S-Function4/1 -> S-Function1/8
  Constant12/1 -> Mux6/1
  Constant11/1 -> Mux6/2
  Mux6/1 -> S-Function1/10, S-Function4/1
  Constant13/1 -> Mux5/1
  Gain/1 -> S-Function1/11
  S-Function5/1 -> Gain/1, S-Function1/12
  Constant14/1 -> S-Function5/1
  Mux7/1 -> S-Function1/6
  From/1 -> Mux2/1
  From1/1 -> Mux2/2
  [Mass] -> Mux10/1
  Extended Kalman Filter2/1 -> Scope14/1, Demux2/1
  S-Function7/1 -> Zero-Order Hold5/1, Plant3/4(liftForce)  "u"
  Constant22/1 -> Mux14/2, Mux11/3, Mux11/2
  Constant19/1 -> S-Function11/1
  Mux13/1 -> S-Function7/10, S-Function10/1
  S-Function7/2 -> Display8/1
  Mux11/1 -> S-Function8/1
  S-Function9/1 -> S-Function7/7
  Constant23/1 -> Mux9/3
  Demux2/3 -> Goto2/1, Scope8/1, Display6/1
  S-Function8/1 -> S-Function7/5
  Mux12/1 -> S-Function7/9, S-Function9/1
  Constant15/1 -> Mux9/2
  Constant18/1 -> Mux12/1
  [Pitch] -> Mux10/2
  Constant20/1 -> S-Function7/4
  Constant16/1 -> Mux13/2
  S-Function11/1 -> Gain1/1, S-Function7/12
  Mux14/1 -> S-Function7/6
  Constant21/1 -> Mux12/2
  Plant3/4(lift_pos) -> Scope12/1, Zero-Order Hold6/1, Derivative2/1, Mux8/1
  Mux8/1 -> S-Function7/2, S-Function7/1
  Mux9/1 -> Extended Kalman Filter2/1, Scope11/1  "inputs"
  Mux10/1 -> S-Function6/1
  Constant17/1 -> Mux13/1
  S-Function6/1 -> S-Function7/3
  Zero-Order Hold6/1 -> Extended Kalman Filter2/2
  S-Function10/1 -> S-Function7/8
  Plant3/3(pitch_angle) -> Display7/1, [Pitch]  "pitch_angle"
  Derivative2/1 -> Mux8/2
  Saturation3/1 -> Mux11/1, Mux14/1, Scope12/2
  Gain1/1 -> S-Function7/11
  Gain2/1 -> S-Function15/11
  Mux15/1 -> S-Function14/1
  Constant25/1 -> Mux18/1
  S-Function14/1 -> S-Function15/3
  S-Function12/1 -> Gain3/1, S-Function15/8
  Mux19/1 -> S-Function15/6
  Constant24/1 -> Mux18/2
  Constant28/1 -> S-Function15/4
  S-Function16/1 -> S-Function15/5
  Constant27/1 -> S-Function13/1
  Mux18/1 -> Gain4/1, S-Function15/10, S-Function12/1
  S-Function15/2 -> Display9/1
  Gain3/1 -> S-Function15/7
  Mux16/1 -> S-Function16/1
  S-Function13/1 -> Gain2/1, S-Function15/12
  Mux20/1 -> Scope18/1, S-Function15/2, S-Function15/1
  Derivative3/1 -> Mux20/2
  Gain4/1 -> S-Function15/9
  Constant26/1 -> Mux9/1
  [Pitch] -> Gain5/1
  Zero-Order Hold/1 -> Extended Kalman Filter3/2
  Mux17/1 -> Extended Kalman Filter3/1
  Zero-Order Hold7/1 -> Mux17/1
  Constant33/1 -> Mux17/2
  Constant34/1 -> Mux17/3
  Demux3/3 -> [rx], Display10/1, Scope19/1
  Extended Kalman Filter3/1 -> Display13/1, Demux3/1
  Constant30/1 -> Mux19/1, Mux16/1, Mux16/3, Mux16/2, Scope15/1, Mux19/2
  S-Function15/1 -> Plant3/5(armTorque), Scope17/1, Zero-Order Hold9/1, Zero-Order Hold7/1  "u"
  Extended Kalman Filter5/1 -> Display11/1, Demux4/1
  Mux21/1 -> Unscented Kalman Filter1/1, Extended Kalman Filter5/1
  Constant32/1 -> Mux21/2
  Constant35/1 -> Mux21/3
  Plant3/5(armPos) -> Scope16/1, Zero-Order Hold8/1, Zero-Order Hold/1, Derivative3/1, Mux20/1
  Zero-Order Hold9/1 -> Mux21/1
  Demux4/3 -> Goto5/1, Scope20/1
  Demux4/4 -> [Mass], Scope21/1
  Ramp3/1 -> Saturation3/1
  [Mass] -> Sum4/1
  Constant29/1 -> Sum4/2
  Constant31/1 -> Mux15/2
  Unscented Kalman Filter1/1 -> Display12/1
  Zero-Order Hold8/1 -> Unscented Kalman Filter1/2, Extended Kalman Filter5/2
  [Mass] -> Mux15/1
